simulink model "model1"  (R2024a)
settings: Solver=VariableStepAuto  StartTime=0.0  StopTime=7  RelTol=1e-8
values from neighbouring files (symbols this model uses):
  a0 = -3.24    [script1.m]
  a1 = 0.0    (= 0)    [script1.m]
settings Model: Creator=eva  LastModifiedBy=eva

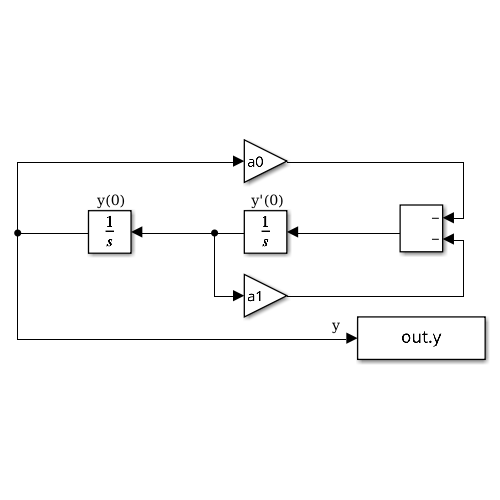
[thumbnail: Simulink's stored preview of the top-level diagram]
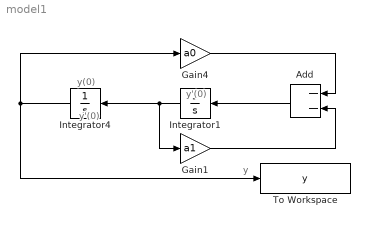
== system model1 ==
  note: y
  note: y'(0)
  note: y'(0)
  note: y(0)
  Add : Sum  Inputs=--
  Gain1 : Gain  Gain=a1
  Gain4 : Gain  Gain=a0
  Integrator1 : Integrator  InitialCondition=0.1
  Integrator4 : Integrator
  To Workspace : ToWorkspace  VariableName=y  SaveFormat=Structure With Time  SampleTime=-1
  wires:
  Integrator1/1 -> Gain1/1, Integrator4/1
  Integrator4/1 -> To Workspace/1, Gain4/1
  Add/1 -> Integrator1/1
  Gain4/1 -> Add/1
  Gain1/1 -> Add/2
